simulink model "msfcndemo_multirate"  (Simulink 7.6)
settings: Solver=ode4  StartTime=0.0  StopTime=25  RelTol=1e-3
values from neighbouring files (symbols this model uses):
  D = [-3    0 ... (first row only)    [csfunc.m]    (also in dsfunc.m = [   -0.8141   -2.9334)
libraries: dspsnks4 x2, dspsigops x1, dspsrcs4 x1
settings Model: Creator=The MathWorks Inc.  ExtModeAutoUpdateStatusClock=off
settings SolverCC: InsertRTBMode=Auto
settings DataIOCC: SaveFormat=Structure  SaveState=on  OutputSaveName=yout1  SignalLoggingName=logsOut
settings OptimizationCC: InitFltsAndDblsToZero=on  BufferReusableBoundary=off
settings DebuggingCC: SaveWithParameterizedLinksMsg=none  SignalResolutionControl=TryResolveAllWithWarning  SolverPrmCheckMsg=none  MultiTaskDSMMsg=warning  MultiTaskCondExecSysMsg=none
settings HardwareCC: TargetEndianess=LittleEndian  TargetHWDeviceType=MATLAB Host  ProdEqTarget=off
settings RTWCC: TLCOptions=-I//sandbox/hfeng/Atest/matlab/test/toolbox/simulink/mlscript  IncludeERTFirstTime=on
settings GRTTargetCC: TargetFcnLib=ansi_tfl_tmw.mat

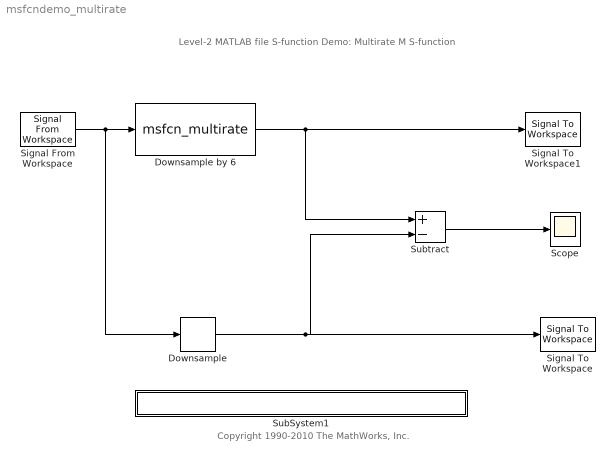
== system msfcndemo_multirate ==
  note: Level-2 MATLAB file S-function Demo:
      | Multirate M S-function
  note: Copyright 1990-2010 The MathWorks, Inc.
  Downsample : dspsigops/Downsample  N=6  phase=5  InputProcessing=Inherited (this choice will be removed - see release notes)  RateOptions=Enforce single-rate processing  smode=Allow multirate  fmode=Maintain input frame rate  ic=0
  Downsample by 6 : M-S-Function  FunctionName=msfcn_multirate
  Scope : Scope
      settings: TimeRange=25  YMin=-1  YMax=1  SampleInput=on
  Signal From Workspace : dspsrcs4/Signal From Workspace  SystemSampleTime=-1  X=1:48  Ts=1  nsamps=1  OutputAfterFinalValue=Setting to zero  ignoreOrWarnInputAndFrameLengths=off
  Signal To Workspace : dspsnks4/Signal To Workspace  SystemSampleTime=-1  VariableName=yout  FrameMode=Concatenate frames (2-D array)
      settings: FixptAsFi=off
  Signal To Workspace1 : dspsnks4/Signal To Workspace  SystemSampleTime=-1  VariableName=yout1  FrameMode=Concatenate frames (2-D array)
      settings: FixptAsFi=off
  SubSystem1 : Subsystem  mask{filename=msfcn_multirate.m}
      mask init:
      | x=sfundemo_maskdisp;
      settings: AttributesFormatString=\n  OpenFcn=sfundemo_openfcn
      mask Display: disp(x);
  Subtract : Sum  Inputs=+-
  wires:
  Downsample/1 -> Signal To Workspace/1, Subtract/2
  Signal From Workspace/1 -> Downsample by 6/1, Downsample/1
  Subtract/1 -> Scope/1
  Downsample by 6/1 -> Signal To Workspace1/1, Subtract/1

== system msfcndemo_multirate/SubSystem1 ==
